simulink model "ECE595_Part1_Project_Lidar_based_Motor_Control_Master"  (R2017a)
settings: Solver=FixedStepDiscrete  StartTime=0.0  StopTime=10.0  FixedStep=0.5  RelTol=1e-3  EnableMultiTasking=on
InitFcn:
  | mbd_s32k14_consistency_checks(bdroot(gcs));
undefined symbols (not defined in the file): B8, C2, C7, D1, D2, F2, G8, G9, H1, H10, H9, J10, J4, J9, K3, PTA0, PTA6, PTA7, PTB0, PTB1, PTC6, PTC7, PTC9, PTD0, PTD6, PTD7, PTE3, PTE4, PTE5, PTE9
libraries: mbd_s32k14_ec_toolbox x7, simulink x1
Description:
  | This model tests FlexCAN communication using CAN with Flexible Data-Rate.
  | The FlexCAN Master sends on each step a message with ID 0x3FF to the slave.
  | On each Tx Complete event Blue LED (PTD0) is toggled.
  | 
  | HW prerequisite:
  | - S32K144EVB-Q100
  | - Make sure that J107 has pin 1 and 2 connected and external power supply is provieded through J16.
  | 
  | Validation:
  | - The CAN Baudrate is set to 500 Kb/s
  | - Any CAN analizer (USB to CAN device) can be used to observe CAN traffic via board CAN port J13.
settings Model: Creator=agrigorev  LastModifiedBy=Akash
settings DataIOCC: ExternalInput=off  InitialState=off  LimitDataPoints=on  SaveFormat=Array  SaveOutput=off  SignalLogging=off  SaveTime=off
settings OptimizationCC: DefaultParameterBehavior=Inlined  LifeSpan=1
settings DebuggingCC: UnderspecifiedInitializationDetection=Classic  MergeDetectMultiDrivingBlocksExec=none  SolverPrmCheckMsg=warning  InheritedTsInSrcMsg=none  SingleTaskRateTransMsg=error  UnconnectedInputMsg=error  UnconnectedOutputMsg=error  UnconnectedLineMsg=error  AllowSymbolicDim=off  UnknownTsInhSupMsg=error  StateNameClashWarn=warning  SFUnexpectedBacktrackingDiag=warning  SFNoUnconditionalDefaultTransitionDiag=warning  SFExecutionAtInitializationDiag=none
settings HardwareCC: ProdBitPerPointer=32  ProdBitPerSizeT=32  ProdBitPerPtrDiffT=32  ProdLargestAtomicInteger=Long  ProdLargestAtomicFloat=Double  ProdIntDivRoundTo=Undefined  ProdWordSize=32  ProdHWDeviceType=ARM Compatible->ARM Cortex
settings ModelReferenceCC: PropagateSignalLabelsOutOfModel=off
settings SFSimCC: MATLABDynamicMemAlloc=off
settings RTWCC: SystemTargetFile=mbd_s32k14.tlc  MakeCommand=mbd_s32k14_make_rtw COPY_MDLREF_INCLUDES=0  TemplateMakefile=mbd_s32k14.tmf  Description=Model Based Design Toolbox S32K14x Code Generation Target
settings CodeAppCC: IgnoreCustomStorageClasses=off
settings STFCustomTargetCC: CombineOutputUpdateFcns=on  ERTCustomFileBanners=on  SupportContinuousTime=off  SupportNonInlinedSFcns=off  RemoveResetFunc=on  MATLABClassNameForMDSCustomization=Simulink.SoftwareTarget.ERTCustomization  GRTInterface=off  SystemTargetFile=mbd_s32k14.tlc
settings ERTTargetCC: MultiwordLength=2048  ParMdlRefBuildCompliant=off  CompOptLevelCompliant=off  ConcurrentExecutionCompliant=off  ERTFirstTimeCompliant=off  ModelStepFunctionPrototypeControlCompliant=off  CPPClassGenCompliant=off  UseToolchainInfoCompliant=off  InlinedParameterPlacement=NonHierarchical  ERTCustomFileTemplate=example_file_process.tlc  ConvertIfToSwitch=off  SuppressUnreachableDefaultCases=off
settings ConfigComp: CovMetricSettings=dw  CovHtmlReporting=on  CovSaveCumulativeToWorkspaceVar=on  CovSaveSingleToWorkspaceVar=on  CovExternalEMLEnable=off

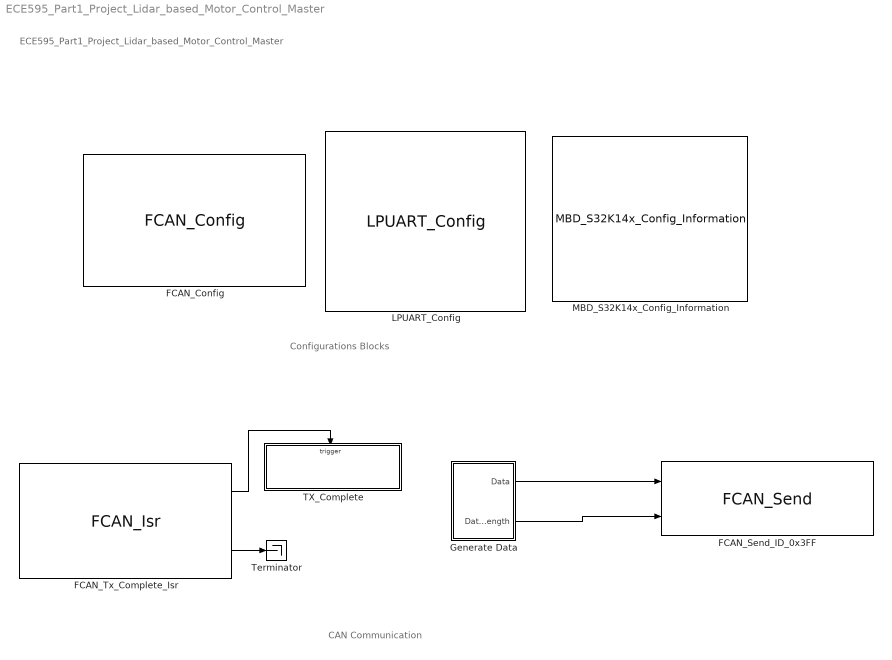
== system ECE595_Part1_Project_Lidar_based_Motor_Control_Master ==
  note: ECE595_Part1_Project_Lidar_based_Motor_Control_Master
  note: CAN Communication
  note: Configurations Blocks
  FCAN_Config : mbd_s32k14_ec_toolbox/S32K14x/Communication Blocks/Flex CAN Blocks/FCAN_Config  Priority=1  can_instance=0  can_mode=Normal mode  can_max_num_mb=16  can_rx=PTE4 : [9] : [6] : [D1]  can_tx=PTE5 : [8] : [5] : [D2]  show_adv_opts=on  can_clk_src=Peripheral clock  can_presdiv=9  can_rjw=0  can_pseg1=3  can_pseg2=3  can_propseg=6  can_cbt_presdiv=9  can_cbt_rjw=0  can_cbt_pseg1=3  can_cbt_pseg2=3  can_cbt_propseg=6  can_fd_enable=on  can_payload=8  can_rxfifo_enable=off  can_fifo_id_filter_extended=off  can_fifo_id_filter_remote=off  can_num_id_filters=8  can_fifo_id_format=A  can_fifo_id_filter={'0x0', '0x0', '0x0', '0x0', '0x0', '0x0', '0x0', '0x0'}  can_pn_enable=off  can_wakeup_match=off  can_wakeup_timeout=off  can_timeout_en=off  can_match_timeout=1  can_multiple_matches_en=off  can_num_matches=1  can_idfilter_extendedid=off  can_idfilter_remoteframe=off  can_idfilter_type=Match exact  can_idfilter_id1=0  can_idfilter_id2=0  can_payloadfilter_enable=off  can_payloadfilter_dlclow=0  can_payloadfilter_dlchigh=0  can_payloadfilter_type=Match exact  can_payloadfilter_payload1_b0=0  can_payloadfilter_payload1_b1=0  can_payloadfilter_payload1_b2=0  can_payloadfilter_payload1_b3=0  can_payloadfilter_payload1_b4=0  can_payloadfilter_payload1_b5=0  can_payloadfilter_payload1_b6=0  can_payloadfilter_payload1_b7=0  can_payloadfilter_payload2_b0=0  can_payloadfilter_payload2_b1=0  can_payloadfilter_payload2_b2=0  can_payloadfilter_payload2_b3=0  can_payloadfilter_payload2_b4=0  can_payloadfilter_payload2_b5=0  can_payloadfilter_payload2_b6=0  can_payloadfilter_payload2_b7=0
  FCAN_Send_ID_0x3FF : mbd_s32k14_ec_toolbox/S32K14x/Communication Blocks/Flex CAN Blocks/FCAN_Send  Priority=2  can_instance=0  can_mode=Non-blocking  can_timeout_ms=0  can_mb_idx=15  can_extended_id=off  can_is_remote=off  can_id=3FF  show_adv_opts=on  can_fd_enable=on  can_enable_brs=off  can_fd_padding=0
  FCAN_Tx_Complete_Isr : mbd_s32k14_ec_toolbox/S32K14x/Communication Blocks/Flex CAN Blocks/FCAN_Isr  can_instance=0  can_event=Tx Complete
  Generate Data : Subsystem
  LPUART_Config : mbd_s32k14_ec_toolbox/S32K14x/Communication Blocks/UART Blocks/LPUART_Config  Priority=2  instance=2  baudrate=115200  databits=8  parity=None  sbns=1  bothedge=rising edge  rxinv=off  txinv=off  show_adv_opts=on  brk13=10 - 13 bit times  lbkde=10 - 13 bit times  rx0=PTB0 : [54] : [34] : [J10]  tx0=PTB1 : [53] : [33] : [J9]  cts0=PTA0 : [79] : [50] : [G8]  rts0=PTC9 : [55] : [35] : [H9]  rx1=PTC6 : [81] : [52] : [C7]  tx1=PTC7 : [80] : [51] : [B8]  cts1=PTA6 : [58] : [38] : [G9]  rts1=PTA7 : [57] : [37] : [H10]  rx2=PTD6 : [32] : [23] : [J4]  tx2=PTD7 : [31] : [22] : [K3]  cts2=PTE9 : [23] : [16] : [H1]  rts2=PTE3 : [18] : [13] : [F2]
  MBD_S32K14x_Config_Information : mbd_s32k14_ec_toolbox/S32K14x/MBD_S32K14x_Config_Information  disp_str=|  config_params=[]
      | Target : S32K144-64KB_SRAM
      | Package : 100-pin
      | System clock : 80 MHz
      | XTAL clock : External 8 MHz
      | Compiler : GCC
      | Target Type : FLASH
      | Download Code after build : (OpenSDA: F)
      | Step Tick Interrupt Priority : 15
  TX_Complete : Subsystem  TreatAsAtomicUnit=on
      settings: RTWSystemCode=Nonreusable function
  Terminator : Terminator
  wires:
  FCAN_Tx_Complete_Isr/1 -> TX_Complete/Trigger
  FCAN_Tx_Complete_Isr/2 -> Terminator/1
  Generate Data/1(Data) -> FCAN_Send_ID_0x3FF/1
  Generate Data/2(Data Length) -> FCAN_Send_ID_0x3FF/2

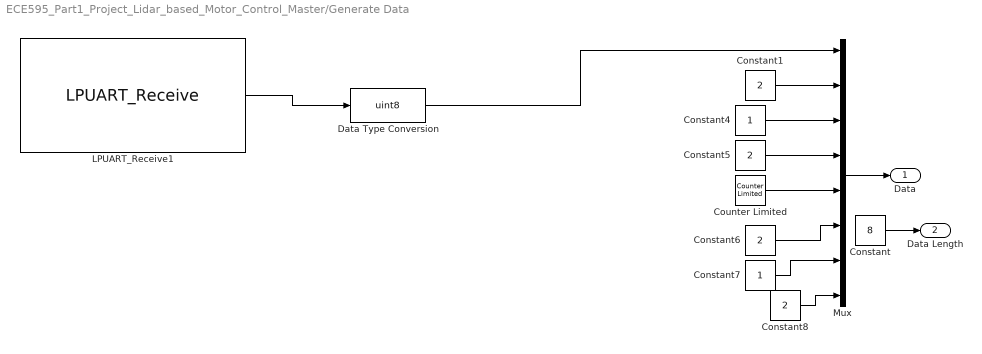
== system ECE595_Part1_Project_Lidar_based_Motor_Control_Master/Generate Data ==
  Constant : Constant  Value=8  OutDataTypeStr=uint8
  Constant{1,5..6,8} (4 alike) : Constant  Value=2  OutDataTypeStr=uint8
  Constant4 : Constant  OutDataTypeStr=uint8
  Constant7 : Constant  OutDataTypeStr=uint8
  Counter Limited : simulink/Sources/Counter Limited  uplimit=255  tsamp=-1
  Data Type Conversion : DataTypeConversion  OutDataTypeStr=uint8
  LPUART_Receive1 : mbd_s32k14_ec_toolbox/S32K14x/Communication Blocks/UART Blocks/LPUART_Receive  instance=2
  Mux : Mux  Inputs=8
  Data : Outport
  Data Length : Outport  Port=2
  wires:
  Constant6/1 -> Mux/6
  Constant4/1 -> Mux/3
  Constant8/1 -> Mux/8
  Constant5/1 -> Mux/4
  Constant/1 -> Data Length/1
  Mux/1 -> Data/1
  Counter Limited/1 -> Mux/5
  Constant7/1 -> Mux/7
  Constant1/1 -> Mux/2
  LPUART_Receive1/1 -> Data Type Conversion/1
  Data Type Conversion/1 -> Mux/1

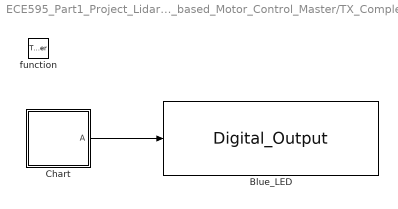
== system ECE595_Part1_Project_Lidar_based_Motor_Control_Master/TX_Complete ==
  function : TriggerPort  TriggerType=function-call  VariantControl=Variant
  Blue_LED : mbd_s32k14_ec_toolbox/S32K14x/Peripheral Interface Blocks/Digital_Output  gpio_pin=PTD0 : [4] : [2] : [C2]  port=D  pin=0  drive_strength=Low  slew_rate=Fast
  Chart : Stateflow chart  TreatAsAtomicUnit=on
  wires:
  Chart/1(" A") -> Blue_LED/1

== stateflow chart ECE595_Part1_Project_Lidar_based_Motor_Control_Master/TX_Complete/Chart ==
  state A
  state A1
  (default) -> A
  A -> A1
  A1 -> A
  data: A output boolean [0..1]
